simulink model "ACCLKS_CarSim"  (Simulink 8.1)
settings: Solver=FixedStepDiscrete  StartTime=0.0  StopTime=200  FixedStep=0.001  RelTol=1e-3
PreLoadFcn:
  | load('Matrix.mat')
  | 
  | Vx = 100;
  | Q1 = 10;
  | Q2 = 5;
  | R = 25;
  | Ts = 0.01;
  | GearRatio = 17.25;
  | 
  | [K,Ad,Bd,Cd,Dd] = dLKS_LQR(Q1,Q2,R,Ts)
undefined symbols (not defined in the file or in its folder): Ad, DiscIntNeverNeededParam, fdesignblkfcn, gcbh, K, sigbuilder_block
libraries: simulink x6, dspadpt3 x1, Solver_SF x1
settings Model: Creator=IVDL_Mola  LastModifiedBy=IVDL
settings DataIOCC: SignalLoggingSaveFormat=Dataset
settings OptimizationCC: ExpressionDepthLimit=128
settings DebuggingCC: FcnCallInpInsideContextMsg=EnableAllAsError  StateNameClashWarn=none
settings GRTTargetCC: CodeReplacementLibrary=None  CombineOutputUpdateFcns=on  CPPClassGenCompliant=on  GRTInterface=off

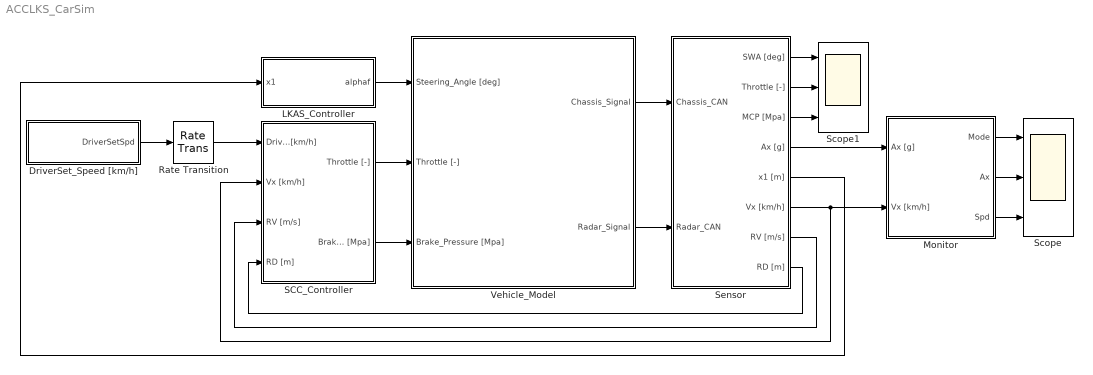
== system ACCLKS_CarSim ==
  DriverSet_Speed [km/h] : Subsystem  Tag=STV Subsys  LoadFcn=sigbuilder_block('load');  StartFcn=sigbuilder_block('start');  StopFcn=sigbuilder_block('stop');  ClipboardFcn=sigbuilder_block('clipboard');  SystemSampleTime=Ts  mask(Sigbuilder block){}
      mask help: Simulink:masks:SigbuilderBlock_MD
      mask init:
      | if ~strcmp(get_param(bdroot(gcbh),'SimulationStatus'),'stopped') tuvar = sigbuilder_block('maskInit'); end
      settings: CopyFcn=sigbuilder_block('copy');  DeleteFcn=sigbuilder_block('delete');  ModelCloseFcn=sigbuilder_block('modelClose');  PreSaveFcn=sigbuilder_block('preSave');  PauseFcn=sigbuilder_block('pause');  ContinueFcn=sigbuilder_block('continue');  NameChangeFcn=sigbuilder_block('namechange');  OpenFcn=sigbuilder_block('open',[361.5 171.75 518.25 401.25 ]);  CloseFcn=sigbuilder_block('close');
      mask Display: plot(0, 0, 100, 100,[2, 2, 32, 32, 2], [68, 8, 8, 68, 68],[32, 2], [38, 38], [32, 19, 2],[53, 60, 44], [32, 17, 17, 2],[16, 16, 31, 31]);txt = getActiveGroup(gcbh);text(2, 100, txt,'verticalAlignment', 'top');
  LKAS_Controller : Subsystem
  Monitor : Subsystem
  Rate Transition : RateTransition
  SCC_Controller : Subsystem
  Scope : Scope  NumInputPorts=3
      settings: ShowLegends=on  TimeRange=200  YMin=-1~-0.001~107.9  YMax=1~0.019~110
  Scope1 : Scope  NumInputPorts=3
      settings: ShowLegends=on  TimeRange=200  YMin=-6~0~0  YMax=6~0.7000000000000001~1.4
  Sensor : Subsystem
  Vehicle_Model : Subsystem
  wires:
  Vehicle_Model/1(Chassis_Signal) -> Sensor/1(Chassis_CAN)
  Vehicle_Model/2(Radar_Signal) -> Sensor/2(Radar_CAN)
  LKAS_Controller/1(alphaf) -> Vehicle_Model/1(Steering_Angle [deg])
  SCC_Controller/2(Brake [Mpa]) -> Vehicle_Model/3(Brake_Pressure [Mpa])
  SCC_Controller/1(Throttle [-]) -> Vehicle_Model/2(Throttle [-])
  Sensor/8(RD [m]) -> SCC_Controller/4(RD [m])
  Sensor/7(RV [m/s]) -> SCC_Controller/3(RV [m/s])
  Sensor/6(Vx [km/h]) -> Monitor/2(Vx [km/h]), SCC_Controller/2(Vx [km/h])
  Sensor/5(x1 [m]) -> LKAS_Controller/1(x1)
  DriverSet_Speed [km/h]/1(DriverSetSpd) -> Rate Transition/1
  Sensor/4(Ax [g]) -> Monitor/1(Ax [g])
  Sensor/3(MCP [Mpa]) -> Scope1/3
  Sensor/2(Throttle [-]) -> Scope1/2
  Sensor/1(SWA [deg]) -> Scope1/1
  Monitor/3(Spd) -> Scope/3
  Monitor/2(Ax) -> Scope/2
  Monitor/1(Mode) -> Scope/1
  Rate Transition/1 -> SCC_Controller/1(Driver_SetSpd [km/h])

== system ACCLKS_CarSim/DriverSet_Speed [km/h] ==
  Demux : Demux  Tag=STV Demux  Outputs=1
  FromWs : FromWorkspace  Tag=STV FromWs  VariableName=tuvar  SampleTime=0  SigBuilderData=DataTag0  VnvData=DataTag1
      SigBuilderData=|
      | common.afterFinalStr = 'Extrapolate'
      | common.sampleTime = 0
      | dataSet.timeRange = [0 100]
      | dataSet.name = 'Group 1'
      | sbobj.Groups.Name = 'Group 1'
      | sbobj.Groups.Signals.Name = 'DriverSetSpd'
      | sbobj.Groups.Signals.XData = [0 25 25 80 80 100]
      | sbobj.Groups.Signals.YData = [70 70 110 110 60 60]
      | sbobj.Groups.TimeRange = [0 100]
  DriverSetSpd : Outport  Tag=STV Outport
  wires:
  FromWs/1 -> Demux/1
  Demux/1 -> DriverSetSpd/1

== system ACCLKS_CarSim/LKAS_Controller ==
  x1 : Inport
  CtrlLaw : Subsystem
  Function-Call Generator : simulink/Ports & Subsystems/Function-Call Generator  sample_time=Ts  numberOfIterations=1
  Function-Call Generator2 : simulink/Ports & Subsystems/Function-Call Generator  sample_time=Ts  numberOfIterations=1
  Observer : Subsystem
  alphaf : Outport
  wires:
  x1/1 -> CtrlLaw/1(x1), Observer/1(x1)
  CtrlLaw/1(alphaf) -> alphaf/1
  Observer/1(x2_hat) -> CtrlLaw/2(x2_hat)
  Observer/2(x3_hat) -> CtrlLaw/3(x3_hat)
  Observer/3(x4_hat) -> CtrlLaw/4(x4_hat)
  Function-Call Generator/1 -> Observer/Trigger
  Function-Call Generator2/1 -> CtrlLaw/Trigger

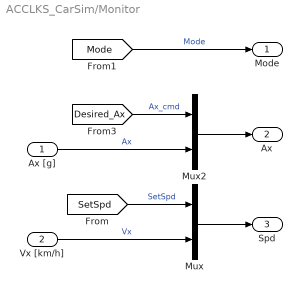
== system ACCLKS_CarSim/Monitor ==
  Ax [g] : Inport
  Vx [km/h] : Inport  Port=2
  Mux : Mux  Inputs=2
  Mux2 : Mux  Inputs=2
  Mode : Outport
  Ax : Outport  Port=2
  Spd : Outport  Port=3
  wires:
  [SetSpd] -> Mux/1  "SetSpd"
  Mux/1 -> Spd/1
  Mux2/1 -> Ax/1
  [Desired_Ax] -> Mux2/1  "Ax_cmd"
  Vx [km/h]/1 -> Mux/2  "Vx"
  [Mode] -> Mode/1  "Mode"
  Ax [g]/1 -> Mux2/2  "Ax"

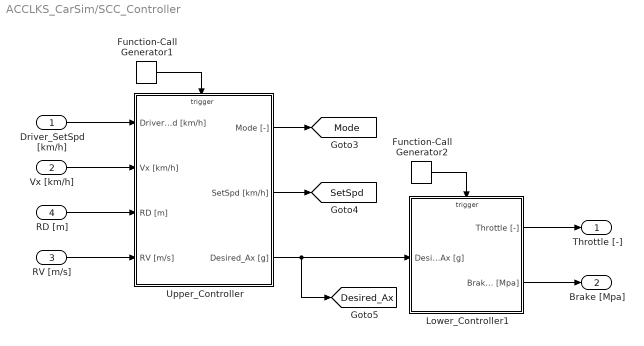
== system ACCLKS_CarSim/SCC_Controller ==
  Driver_SetSpd [km/h] : Inport
  Vx [km/h] : Inport  Port=2
  RV [m/s] : Inport  Port=3
  RD [m] : Inport  Port=4
  Function-Call Generator1 : simulink/Ports & Subsystems/Function-Call Generator  sample_time=Ts  numberOfIterations=1
  Function-Call Generator2 : simulink/Ports & Subsystems/Function-Call Generator  sample_time=Ts  numberOfIterations=1
  Lower_Controller1 : Subsystem
  Upper_Controller : Subsystem
  Throttle [-] : Outport
  Brake [Mpa] : Outport  Port=2
  tag scope: Desired_Ax=global, Mode=global, SetSpd=global
  wires:
  Driver_SetSpd [km/h]/1 -> Upper_Controller/1(Driver_SetSpd [km/h])
  Lower_Controller1/2(Brake [Mpa]) -> Brake [Mpa]/1
  Lower_Controller1/1(Throttle [-]) -> Throttle [-]/1
  RD [m]/1 -> Upper_Controller/3(RD [m])
  Vx [km/h]/1 -> Upper_Controller/2(Vx [km/h])
  RV [m/s]/1 -> Upper_Controller/4(RV [m/s])
  Upper_Controller/3(Desired_Ax [g]) -> Lower_Controller1/1(Desired_Ax [g]), [Desired_Ax]
  Upper_Controller/1(Mode [-]) -> [Mode]
  Upper_Controller/2(SetSpd [km/h]) -> [SetSpd]
  Function-Call Generator1/1 -> Upper_Controller/Trigger
  Function-Call Generator2/1 -> Lower_Controller1/Trigger

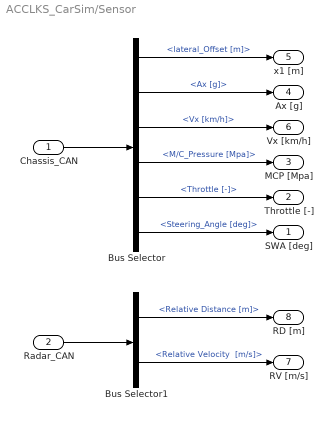
== system ACCLKS_CarSim/Sensor ==
  Chassis_CAN : Inport
  Radar_CAN : Inport  Port=2
  Bus Selector : BusSelector  OutputSignals=lateral_Offset [m],Ax [g],Vx [km/h],M/C_Pressure [Mpa],Throttle [-],Steering_Angle [deg]
  Bus Selector1 : BusSelector  OutputSignals="Relative Distance [m],Relative Velocity  [m/s]"
  SWA [deg] : Outport
  Throttle [-] : Outport  Port=2
  MCP [Mpa] : Outport  Port=3
  Ax [g] : Outport  Port=4
  x1 [m] : Outport  Port=5
  Vx [km/h] : Outport  Port=6
  RV [m/s] : Outport  Port=7
  RD [m] : Outport  Port=8
  wires:
  Bus Selector/3 -> Vx [km/h]/1  "<Vx [km/h]>"
  Bus Selector/2 -> Ax [g]/1  "<Ax [g]>"
  Chassis_CAN/1 -> Bus Selector/1
  Bus Selector/4 -> MCP [Mpa]/1  "<M/C_Pressure [Mpa]>"
  Bus Selector/5 -> Throttle [-]/1  "<Throttle [-]>"
  Bus Selector/1 -> x1 [m]/1  "<lateral_Offset [m]>"
  Bus Selector/6 -> SWA [deg]/1  "<Steering_Angle [deg]>"
  Bus Selector1/1 -> RD [m]/1  "<Relative Distance [m]>"
  Bus Selector1/2 -> RV [m/s]/1  "<Relative Velocity  [m/s]>"
  Radar_CAN/1 -> Bus Selector1/1

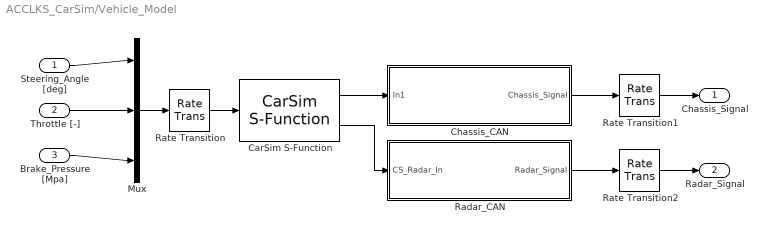
== system ACCLKS_CarSim/Vehicle_Model ==
  Steering_Angle [deg] : Inport
  Throttle [-] : Inport  Port=2
  Brake_Pressure [Mpa] : Inport  Port=3
  CarSim S-Function : Solver_SF/CarSim S-Function  Priority=1  VehicleCode=i_i  SIMFILE=simfile
  Chassis_CAN : Subsystem
  Mux : Mux  Inputs=3
  Radar_CAN : Subsystem
  Rate Transition : RateTransition
  Rate Transition1 : RateTransition
  Rate Transition2 : RateTransition
  Chassis_Signal : Outport
  Radar_Signal : Outport  Port=2
  wires:
  CarSim S-Function/2 -> Radar_CAN/1(CS_Radar_In)
  CarSim S-Function/1 -> Chassis_CAN/1(In1)
  Radar_CAN/1(Radar_Signal) -> Rate Transition2/1
  Rate Transition1/1 -> Chassis_Signal/1
  Rate Transition2/1 -> Radar_Signal/1
  Throttle [-]/1 -> Mux/2
  Brake_Pressure [Mpa]/1 -> Mux/3
  Chassis_CAN/1(Chassis_Signal) -> Rate Transition1/1
  Mux/1 -> Rate Transition/1
  Rate Transition/1 -> CarSim S-Function/1
  Steering_Angle [deg]/1 -> Mux/1

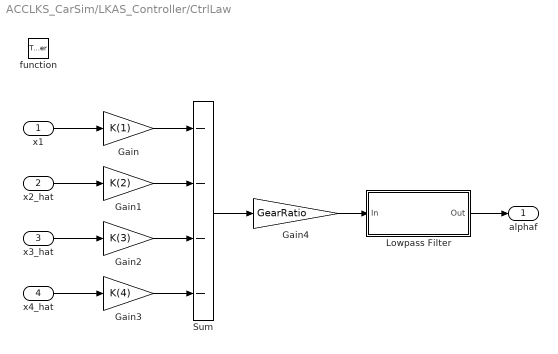
== system ACCLKS_CarSim/LKAS_Controller/CtrlLaw ==
  x1 : Inport
  x2_hat : Inport  Port=2
  x3_hat : Inport  Port=3
  x4_hat : Inport  Port=4
  function : TriggerPort  TriggerType=function-call  SampleTime=-1
  Gain : Gain  Gain=K(1)  OutDataTypeStr=double
  Gain1 : Gain  Gain=K(2)
  Gain2 : Gain  Gain=K(3)
  Gain3 : Gain  Gain=K(4)
  Gain4 : Gain  Gain=GearRatio  OutDataTypeStr=double
  Lowpass Filter : Subsystem  DialogController=fdesignblkfcn  DialogControllerArgs=DataTag3  InitFcn=fdesignblkfcn(gcbh, {'InitFcn'});  mask(Lowpass Filter){}
      mask help: Design a lowpass filter
      settings: CopyFcn=fdesignblkfcn(gcbh, {'CopyFcn'});
      mask Help: helpview(mapfilelocation('dsp'), 'dsplowpassfilter');
      mask Display: disp('Lowpass')
  Sum : Sum  Inputs=----  AccumDataTypeStr=double
  alphaf : Outport  OutDataTypeStr=double
  wires:
  x1/1 -> Gain/1
  Gain/1 -> Sum/1
  Gain1/1 -> Sum/2
  Gain3/1 -> Sum/4
  Gain2/1 -> Sum/3
  Sum/1 -> Gain4/1
  x2_hat/1 -> Gain1/1
  x3_hat/1 -> Gain2/1
  x4_hat/1 -> Gain3/1
  Gain4/1 -> Lowpass Filter/1(In)
  Lowpass Filter/1(Out) -> alphaf/1

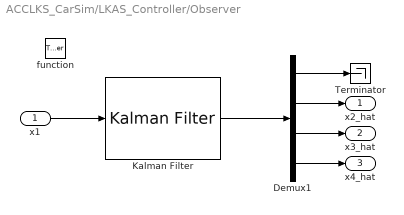
== system ACCLKS_CarSim/LKAS_Controller/Observer ==
  x1 : Inport
  function : TriggerPort  TriggerType=function-call  SampleTime=-1
  Demux1 : Demux
  Kalman Filter : dspadpt3/Kalman Filter  num_targets=1  sourceEnable=Always  isReset=on  X=zeros([4, 1])  P=10*eye(4)  A=Ad  sourceMeasure=Specify via Dialog  H=Cd  Q=0.05*eye(4)  R=eye(1)  isOutputEstMeasure=off  isOutputEstState=on  isOutputEstError=off  isOutputPrdMeasure=off  isOutputPrdState=off  isOutputPrdError=off
  Terminator : Terminator
  x2_hat : Outport
  x3_hat : Outport  Port=2
  x4_hat : Outport  Port=3
  wires:
  Demux1/3 -> x3_hat/1
  Demux1/1 -> Terminator/1
  Kalman Filter/1 -> Demux1/1
  x1/1 -> Kalman Filter/1
  Demux1/2 -> x2_hat/1
  Demux1/4 -> x4_hat/1

== system ACCLKS_CarSim/SCC_Controller/Lower_Controller1 ==
  Desired_Ax [g] : Inport
  function : TriggerPort  TriggerType=function-call
  Brake_Controller : Subsystem
  Throttle_Controller : Subsystem
  Throttle [-] : Outport
  Brake [Mpa] : Outport  Port=2
  wires:
  Desired_Ax [g]/1 -> Brake_Controller/1(Desired_Ax [g]), Throttle_Controller/1(Desired_Ax [g])
  Throttle_Controller/1(Throttle [-]) -> Throttle [-]/1
  Brake_Controller/1(Brake [Mpa]) -> Brake [Mpa]/1

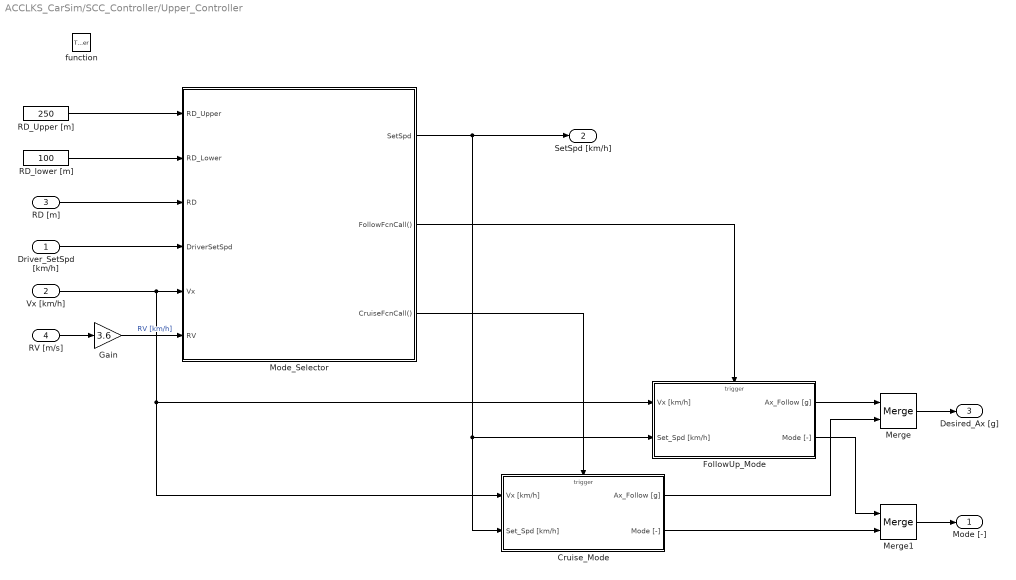
== system ACCLKS_CarSim/SCC_Controller/Upper_Controller ==
  Driver_SetSpd [km/h] : Inport
  Vx [km/h] : Inport  Port=2
  RD [m] : Inport  Port=3
  RV [m/s] : Inport  Port=4
  function : TriggerPort  TriggerType=function-call
  Cruise_Mode : Subsystem  TreatAsAtomicUnit=on
  FollowUp_Mode : Subsystem  TreatAsAtomicUnit=on
  Gain : Gain  Gain=3.6
  Merge : Merge
  Merge1 : Merge
  Mode_Selector : Stateflow chart  TreatAsAtomicUnit=on
  RD_Upper [m] : Constant  Value=250
  RD_lower [m] : Constant  Value=100
  Mode [-] : Outport
  SetSpd [km/h] : Outport  Port=2
  Desired_Ax [g] : Outport  Port=3
  wires:
  RD_lower [m]/1 -> Mode_Selector/2(RD_Lower)
  RD_Upper [m]/1 -> Mode_Selector/1(RD_Upper)
  Driver_SetSpd [km/h]/1 -> Mode_Selector/4(DriverSetSpd)
  RD [m]/1 -> Mode_Selector/3(RD)
  Vx [km/h]/1 -> FollowUp_Mode/1(Vx [km/h]), Cruise_Mode/1(Vx [km/h]), Mode_Selector/5(Vx)
  RV [m/s]/1 -> Gain/1
  Gain/1 -> Mode_Selector/6(RV)  "RV [km/h]"
  Cruise_Mode/1(Ax_Follow [g]) -> Merge/2
  FollowUp_Mode/2(Mode [-]) -> Merge1/1
  Cruise_Mode/2(Mode [-]) -> Merge1/2
  Merge/1 -> Desired_Ax [g]/1
  Merge1/1 -> Mode [-]/1
  Mode_Selector/1(SetSpd) -> Cruise_Mode/2(Set_Spd [km/h]), FollowUp_Mode/2(Set_Spd [km/h]), SetSpd [km/h]/1
  Mode_Selector/2(FollowFcnCall()) -> FollowUp_Mode/Trigger
  Mode_Selector/3(CruiseFcnCall()) -> Cruise_Mode/Trigger
  FollowUp_Mode/1(Ax_Follow [g]) -> Merge/1

== system ACCLKS_CarSim/Vehicle_Model/Chassis_CAN ==
  In1 : Inport
  Bus Creator : BusCreator  Inputs=6
  Demux1 : Demux  Outputs=6
  Chassis_Signal : Outport
  wires:
  In1/1 -> Demux1/1
  Demux1/1 -> Bus Creator/1  "lateral_Offset [m]"
  Demux1/2 -> Bus Creator/2  "Ax [g]"
  Demux1/3 -> Bus Creator/3  "Vx [km/h]"
  Demux1/4 -> Bus Creator/4  "M/C_Pressure [Mpa]"
  Demux1/5 -> Bus Creator/5  "Throttle [-]"
  Demux1/6 -> Bus Creator/6  "Steering_Angle [deg]"
  Bus Creator/1 -> Chassis_Signal/1

== system ACCLKS_CarSim/Vehicle_Model/Radar_CAN ==
  CS_Radar_In : Inport
  Bus Creator1 : BusCreator  Inputs=11
  Demux1 : Demux  Outputs=11
  Radar_Signal : Outport
  wires:
  Bus Creator1/1 -> Radar_Signal/1
  CS_Radar_In/1 -> Demux1/1
  Demux1/9 -> Bus Creator1/9  "Els [rad]"
  Demux1/5 -> Bus Creator1/5  "Width [m]"
  Demux1/11 -> Bus Creator1/11  "Pitch Angle [rad]"
  Demux1/10 -> Bus Creator1/10  "Yaw Angle [rad]"
  Demux1/6 -> Bus Creator1/6  "BrCS [rad]"
  Demux1/7 -> Bus Creator1/7  "BrLS [rad]"
  Demux1/4 -> Bus Creator1/4  "Magnitude [-]"
  Demux1/8 -> Bus Creator1/8  "BrRS [rad]"
  Demux1/1 -> Bus Creator1/1  "Sensor_ID [-]"
  Demux1/2 -> Bus Creator1/2  "Relative Distance [m]"
  Demux1/3 -> Bus Creator1/3  "Relative Velocity  [m/s]"

== system ACCLKS_CarSim/LKAS_Controller/CtrlLaw/Lowpass Filter ==
  In : Inport
  Generated Filter Block : DiscreteFir  Tag=BlockMethodSubSystem  Coefficients=[-0.12703898269324654 0.60128910085241971 0.60128910085241971 -0.12703898269324654]  InputProcessing=Columns as channels (frame based)
  Out : Outport
  wires:
  In/1 -> Generated Filter Block/1
  Generated Filter Block/1 -> Out/1

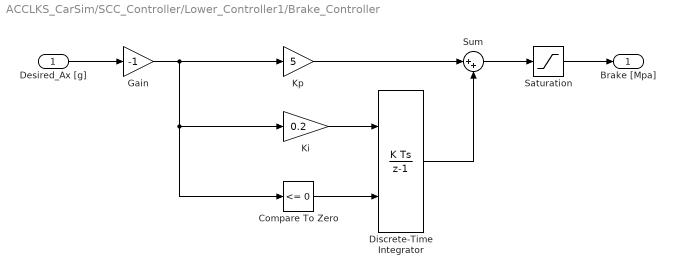
== system ACCLKS_CarSim/SCC_Controller/Lower_Controller1/Brake_Controller ==
  Desired_Ax [g] : Inport
  Compare To Zero : simulink/Logic and Bit Operations/Compare To Zero  relop=<=  OutDataTypeStr=boolean
  Discrete-Time Integrator : DiscreteIntegrator  ExternalReset=rising  SampleTime=-1  ICPrevOutput=DiscIntNeverNeededParam  ICPrevScaledInput=DiscIntNeverNeededParam
  Gain : Gain  Gain=-1
  Ki : Gain  Gain=0.2
  Kp : Gain  Gain=5
  Saturation : Saturate  UpperLimit=6  LowerLimit=0
  Sum : Sum  Inputs=|++
  Brake [Mpa] : Outport
  wires:
  Sum/1 -> Saturation/1
  Saturation/1 -> Brake [Mpa]/1
  Desired_Ax [g]/1 -> Gain/1
  Kp/1 -> Sum/1
  Ki/1 -> Discrete-Time Integrator/1
  Discrete-Time Integrator/1 -> Sum/2
  Gain/1 -> Compare To Zero/1, Ki/1, Kp/1
  Compare To Zero/1 -> Discrete-Time Integrator/2

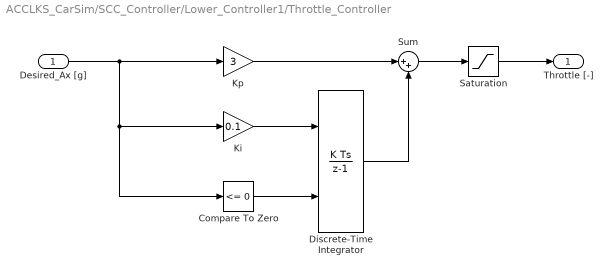
== system ACCLKS_CarSim/SCC_Controller/Lower_Controller1/Throttle_Controller ==
  Desired_Ax [g] : Inport
  Compare To Zero : simulink/Logic and Bit Operations/Compare To Zero  relop=<=  OutDataTypeStr=boolean
  Discrete-Time Integrator : DiscreteIntegrator  ExternalReset=rising  SampleTime=-1  ICPrevOutput=DiscIntNeverNeededParam  ICPrevScaledInput=DiscIntNeverNeededParam
  Ki : Gain  Gain=0.1
  Kp : Gain  Gain=3
  Saturation : Saturate  UpperLimit=0.7  LowerLimit=0
  Sum : Sum  Inputs=|++
  Throttle [-] : Outport
  wires:
  Sum/1 -> Saturation/1
  Saturation/1 -> Throttle [-]/1
  Desired_Ax [g]/1 -> Compare To Zero/1, Ki/1, Kp/1
  Kp/1 -> Sum/1
  Ki/1 -> Discrete-Time Integrator/1
  Compare To Zero/1 -> Discrete-Time Integrator/2
  Discrete-Time Integrator/1 -> Sum/2

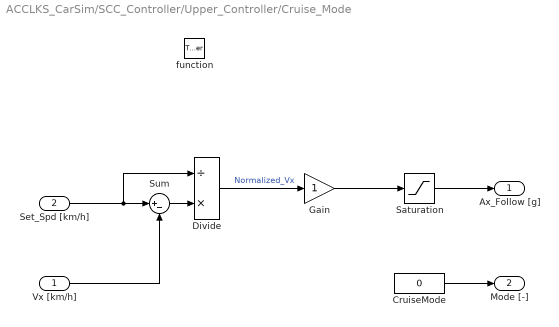
== system ACCLKS_CarSim/SCC_Controller/Upper_Controller/Cruise_Mode ==
  Vx [km/h] : Inport
  Set_Spd [km/h] : Inport  Port=2
  function : TriggerPort  TriggerType=function-call
  CruiseMode : Constant  Value=0
  Divide : Product  Inputs=/*
  Gain : Gain
  Saturation : Saturate  UpperLimit=0.3  LowerLimit=-0.3
  Sum : Sum  Inputs=|+-
  Ax_Follow [g] : Outport
  Mode [-] : Outport  Port=2
  wires:
  Set_Spd [km/h]/1 -> Divide/1, Sum/1
  Vx [km/h]/1 -> Sum/2
  Sum/1 -> Divide/2
  Divide/1 -> Gain/1  "Normalized_Vx"
  Gain/1 -> Saturation/1
  Saturation/1 -> Ax_Follow [g]/1
  CruiseMode/1 -> Mode [-]/1

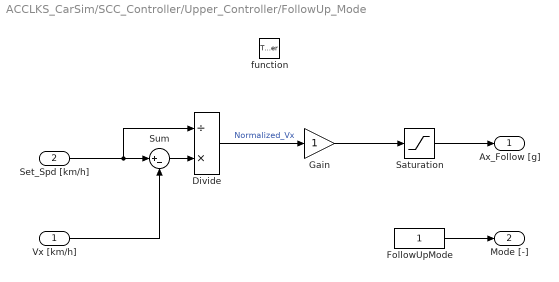
== system ACCLKS_CarSim/SCC_Controller/Upper_Controller/FollowUp_Mode ==
  Vx [km/h] : Inport
  Set_Spd [km/h] : Inport  Port=2
  function : TriggerPort  TriggerType=function-call
  Divide : Product  Inputs=/*
  FollowUpMode : Constant
  Gain : Gain
  Saturation : Saturate  UpperLimit=0.4  LowerLimit=-0.4
  Sum : Sum  Inputs=|+-
  Ax_Follow [g] : Outport
  Mode [-] : Outport  Port=2
  wires:
  Set_Spd [km/h]/1 -> Divide/1, Sum/1
  Vx [km/h]/1 -> Sum/2
  Sum/1 -> Divide/2
  Divide/1 -> Gain/1  "Normalized_Vx"
  Gain/1 -> Saturation/1
  Saturation/1 -> Ax_Follow [g]/1
  FollowUpMode/1 -> Mode [-]/1

== stateflow chart SCC_Controller/Upper_Controller/Mode_Selector ==
  state Cruise_Mode
    du, en : TVSpd = RV+Vx;
    du : send(CruiseFcnCall)
    du : SetSpd = DriverSetSpd;
  state FollowUp_Mode
    du, en : TVSpd = RV+Vx;
    du : send(FollowFcnCall)
    du : SetSpd = TVSpd;
  (default) -> Cruise_Mode
  Cruise_Mode -> FollowUp_Mode : [(RD<=RD_Lower) & (DriverSetSpd >= TVSpd)]
  FollowUp_Mode -> Cruise_Mode : [(RD>RD_Upper) | (DriverSetSpd < TVSpd)]
  data: RD_Upper input double; RD_Lower input double; RD input double; DriverSetSpd input double; SetSpd output double; Vx input double; RV input double; TVSpd local double
  events: FollowFcnCall output FUNCTION_CALL_EVENT; CruiseFcnCall output FUNCTION_CALL_EVENT
